simulink model "mcb_microchip_pmsm_autotuner_SAME70"  (R2023a)
settings: Solver=FixedStepDiscrete  StartTime=0.0  StopTime=30  RelTol=1e-3  EnableMultiTasking=on
InitFcn:
  | mcb_microchip_pmsm_autotuner_SAME70_data;
values from neighbouring files (symbols this model uses):
  PU_System = mcb_SetPUSystem(pmsm,inverter)    [mcb_microchip_pmsm_autotuner_SAME70_data.m]
  Ts = T_pwm    (= 5e-05)    [mcb_microchip_pmsm_autotuner_SAME70_data.m]
  Ts_motor = T_pwm/2    (= 2.5e-05)    [mcb_microchip_pmsm_autotuner_SAME70_data.m]
  Ts_simulink = T_pwm/2    (= 2.5e-05)    [mcb_microchip_pmsm_autotuner_SAME70_data.m]
  Ts_speed = 2 * Ts    (= 0.0001)    [mcb_microchip_pmsm_autotuner_SAME70_data.m]
undefined symbols (not defined in the file or in its folder): A24, AD10, AD7, inverter, LQFP144, MaxPer, ms, ns, PA0, PA1, PA10, PA11, PA12, PA13, PA16, PA18, PA9, PB0, PD18, PD19, PD24, PD25, PD26, PI_params, Pin, pmsm, Resol, SAME70Q21B, target, Timer, Unsigned
libraries: simulink x13, MCHP_Blockset x13, mcbcontrolslib x7, slpidlib x3, mcbpositiondecoderlib x3, svdutilitieslib x3, mcbplantlib x1, autolibpmsmexterior x1, focautotunershared x1
(part 3 of 4)

== system mcb_microchip_pmsm_autotuner_SAME70/Microcontroller/Heartbeat LED ==
  Codegen : Subsystem  VariantControl=(codegen)
  Sim : Subsystem  VariantControl=(sim)

== system mcb_microchip_pmsm_autotuner_SAME70/Microcontroller/Input HW Drivers ==
  PhaseCurr_fb : Inport
  Position_fb : Inport  Port=2
  Codegen : Subsystem  VariantControl=(codegen)
  Sim : Subsystem  VariantControl=(sim)
  IabADC : Outport
  VdcADC : Outport  Port=2
  Vabc_ADC : Outport  Port=3
  eQEP : Outport  Port=4

== system mcb_microchip_pmsm_autotuner_SAME70/Microcontroller/Input Scaling ==
  Mode : Inport
  Iab_ADC : Inport  Port=2
  Vdc_ADC : Inport  Port=3
  Vabc_ADC : Inport  Port=4
  Gain : Gain  Gain=inverter.VoltPerCount  OutDataTypeStr=dataType  RndMeth=Simplest
  Gain1 : Gain  Gain=inverter.VoltPerCount  OutDataTypeStr=dataType  RndMeth=Simplest
  Variant Subsystem : Subsystem  Variant=on
  Iab : Outport
  Vdc : Outport  Port=2
  Vabc : Outport  Port=3
  wires:
  Variant Subsystem/1(Iab) -> Iab/1
  Mode/1 -> Variant Subsystem/1(Mode)
  Iab_ADC/1 -> Variant Subsystem/2(Iab_ADC)
  Vdc_ADC/1 -> Gain/1
  Gain/1 -> Vdc/1
  Vabc_ADC/1 -> Gain1/1
  Gain1/1 -> Vabc/1

== system mcb_microchip_pmsm_autotuner_SAME70/Microcontroller/Mode Control ==
  ClosedLoop : Subsystem  VariantControl=inverter.ADCOffsetCalibEnable == 0 && pmsm.QEPIndexPresent == true
  CurrentCalib : Subsystem  VariantControl=inverter.ADCOffsetCalibEnable == 1 && pmsm.QEPIndexPresent == true
  CurrentPosCalib : Subsystem  VariantControl=inverter.ADCOffsetCalibEnable == 1 && pmsm.QEPIndexPresent == false
  PosCalib : Subsystem  VariantControl=inverter.ADCOffsetCalibEnable == 0 && pmsm.QEPIndexPresent == false
  Mode : Outport

== system mcb_microchip_pmsm_autotuner_SAME70/Microcontroller/Output PWM Drivers ==
  PWM_In : Inport
  InvEn : Inport  Port=2
  Codegen : Subsystem  VariantControl=(codegen)
  Sim : Subsystem  VariantControl=(sim)
  PWM : Outport

== system mcb_microchip_pmsm_autotuner_SAME70/Microcontroller/Output Scaling ==
  Mode : Inport
  Vabc_Ref : Inport  Port=2
  InverterEn : Inport  Port=3
  Constant2 : Constant  OutDataTypeStr=dataType
  Current offset measurement : Constant  Value=[0 0 0]  OutDataTypeStr=dataType
  Mode1 : InportShadow
  Mode2 : InportShadow
  Position offset calibration : Constant  Value=[0.2 -0.1 -0.1]  OutDataTypeStr=dataType
  Switch : Switch  Threshold=1  SaturateOnIntegerOverflow=off  InputSameDT=off
  Switch1 : Switch  Threshold=2  SaturateOnIntegerOverflow=off  InputSameDT=off
  Switch2 : Switch  Threshold=2  SaturateOnIntegerOverflow=off  InputSameDT=off
  PWM : Outport
  InvEn : Outport  Port=2
  wires:
  Switch/1 -> PWM/1
  Switch1/1 -> InvEn/1
  Mode/1 -> Switch/2
  Current offset measurement/1 -> Switch/3
  Switch2/1 -> Switch/1
  Mode1/1 -> Switch2/2
  Vabc_Ref/1 -> Switch2/1
  Position offset calibration/1 -> Switch2/3
  InverterEn/1 -> Switch1/1
  Mode2/1 -> Switch1/2
  Constant2/1 -> Switch1/3

== system mcb_microchip_pmsm_autotuner_SAME70/Microcontroller/SCI In Abstraction ==
  SCI_Data : Inport
  Mode : Inport  Port=2
  Variant Subsystem : Subsystem  Variant=on  VariantControlMode=sim codegen switching
  ConfigAndCommand : Outport
  DebugSel : Outport  Port=2
  wires:
  Variant Subsystem/1(ConfigAndCommand) -> ConfigAndCommand/1
  Variant Subsystem/2(DebugSel) -> DebugSel/1
  SCI_Data/1 -> Variant Subsystem/1(SCI_Data)
  Mode/1 -> Variant Subsystem/2(Mode)

== system mcb_microchip_pmsm_autotuner_SAME70/Microcontroller/SCI Out Abstraction ==
  DebugSel : Inport
  DebugData : Inport  Port=2
  Bus Selector : BusSelector  OutputSignals=PI Params.daxis_gains.P,PI Params.daxis_gains.I,PI Params.qaxis_gains.P,PI Params.qaxis_gains.I,PI Params.speed_gains.P,PI Params.speed_gains.I
  Bus Selector1 : BusSelector  OutputSignals=SpeedFb,Iab,Theta
  Byte Pack : svdutilitieslib/Byte Pack  maskPackedDataType=uint8  datatypes={'single'}  byteAlign=1  blockPlatform=tic2000
  Byte Pack1 : svdutilitieslib/Byte Pack  maskPackedDataType=uint8  datatypes={'single'}  byteAlign=1  blockPlatform=tic2000
  Byte Pack2 : svdutilitieslib/Byte Pack  maskPackedDataType=uint8  datatypes={'single'}  byteAlign=1  blockPlatform=tic2000
  Constant : Constant  Value=0  OutDataTypeStr=dataType
  Counter Free-Running : simulink/Sources/Counter Free-Running  NumBits=3  tsamp=0.5
  Data Type Conversion : DataTypeConversion  OutDataTypeStr=single  RndMeth=Simplest  SaturateOnIntegerOverflow=off
  Demux : Demux  Outputs=2
  Multiport Switch : MultiPortSwitch  Inputs=7  DiagnosticForDefault=None  SaturateOnIntegerOverflow=off  InputSameDT=off
  Multiport Switch1 : MultiPortSwitch  Inputs=4  DiagnosticForDefault=None  SaturateOnIntegerOverflow=off  InputSameDT=off
  Mux : Mux  Inputs=3
  Rate Transition2 : RateTransition  Deterministic=off  OutPortSampleTime=Ts
  DebugSignal : Outport
  wires:
  Counter Free-Running/1 -> Data Type Conversion/1
  Data Type Conversion/1 -> Rate Transition2/1
  DebugData/1 -> Bus Selector1/1, Bus Selector/1
  Bus Selector/4 -> Multiport Switch/5  "<I>"
  Bus Selector/5 -> Multiport Switch/6  "<P>"
  Bus Selector/3 -> Multiport Switch/4  "<P>"
  Bus Selector/6 -> Multiport Switch/7  "<I>"
  Bus Selector/2 -> Multiport Switch/3  "<I>"
  Bus Selector/1 -> Multiport Switch/2  "<P>"
  Constant/1 -> Multiport Switch/8
  DebugSel/1 -> Multiport Switch1/1
  Multiport Switch/1 -> Byte Pack/1
  Multiport Switch1/1 -> Byte Pack1/1
  Bus Selector1/1 -> Multiport Switch1/2  "<SpeedFb>"
  Bus Selector1/3 -> Multiport Switch1/5  "<Theta>"
  Bus Selector1/2 -> Demux/1  "<Iab>"
  Demux/1 -> Multiport Switch1/3
  Demux/2 -> Multiport Switch1/4
  Mux/1 -> DebugSignal/1
  Rate Transition2/1 -> Multiport Switch/1, Byte Pack2/1
  Byte Pack/1 -> Mux/2
  Byte Pack1/1 -> Mux/3
  Byte Pack2/1 -> Mux/1

== system mcb_microchip_pmsm_autotuner_SAME70/Microcontroller/SCI_Rx ==
  CodeGen : Subsystem
  Sim : Subsystem
  Variant Source : VariantSource  VariantControlMode=sim codegen switching
  Data : Outport
  wires:
  CodeGen/1(Data) -> Variant Source/1
  Variant Source/1 -> Data/1
  Sim/1(Data) -> Variant Source/2

== system mcb_microchip_pmsm_autotuner_SAME70/Microcontroller/SCI_Tx ==
  SCI_Tx_Data : Inport
  Codegen : Subsystem  SystemSampleTime=0.03  VariantControl=(codegen)
  Sim : Subsystem  VariantControl=(sim)

== system mcb_microchip_pmsm_autotuner_SAME70/Inverter and Motor/Inverter and Motor/Codegen ==
  Duty_Cycles : Inport
  Ground : Ground
  Terminator : Terminator
  PhaseCurr_fb : Outport
  Position_fb : Outport  Port=2
  wires:
  Duty_Cycles/1 -> Terminator/1
  Ground/1 -> PhaseCurr_fb/1, Position_fb/1

== system mcb_microchip_pmsm_autotuner_SAME70/Inverter and Motor/Inverter and Motor/Sim ==
  Duty_Cycles : Inport
  Motor : Subsystem
  RT1 : RateTransition  Deterministic=off  OutPortSampleTime=Ts_simulink
  RT2 : RateTransition  Deterministic=off  OutPortSampleTime=Ts_simulink
  Rate Transition2 : RateTransition  Deterministic=off  OutPortSampleTime=Ts
  Rate Transition3 : RateTransition  Deterministic=off  OutPortSampleTime=Ts_inverter
  Rate Transition4 : RateTransition  Deterministic=off  OutPortSampleTime=Ts
  Sensor Measurements : Subsystem
  PhaseCurr_fb : Outport
  Position_fb : Outport  Port=2
  wires:
  RT1/1 -> Sensor Measurements/2(PhaseCurr)
  Duty_Cycles/1 -> Rate Transition3/1
  Sensor Measurements/2(Position_fb) -> Rate Transition4/1
  Sensor Measurements/1(PhaseCurr_fb) -> Rate Transition2/1
  Rate Transition2/1 -> PhaseCurr_fb/1
  Rate Transition4/1 -> Position_fb/1
  RT2/1 -> Sensor Measurements/1(Info)
  Rate Transition3/1 -> Motor/1(Duty_Cycles)
  Motor/1(ThetaMech) -> RT2/1
  Motor/2(Iabc) -> RT1/1

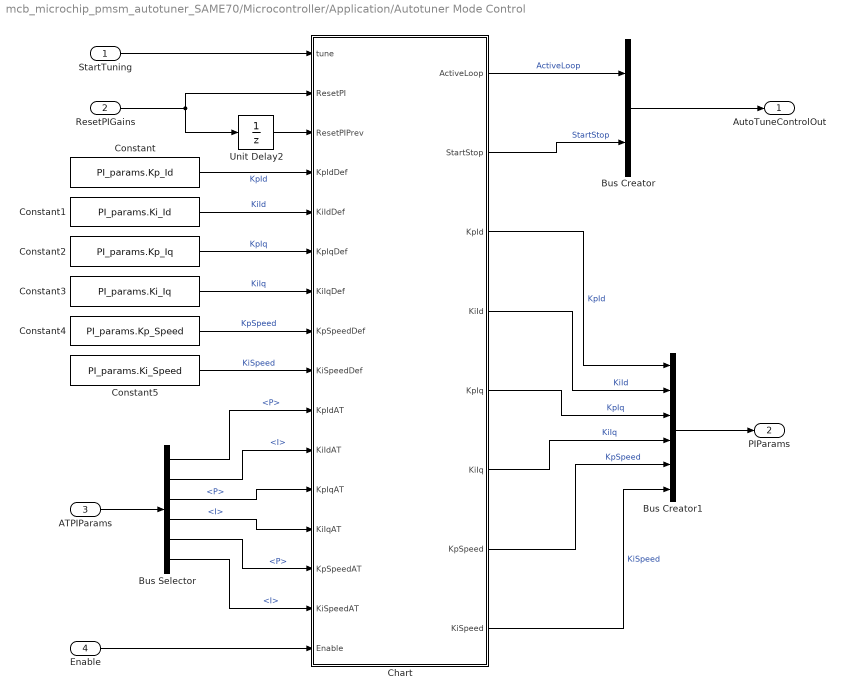
== system mcb_microchip_pmsm_autotuner_SAME70/Microcontroller/Application/Autotuner Mode Control ==
  StartTuning : Inport
  ResetPIGains : Inport  Port=2
  ATPIParams : Inport  Port=3
  Enable : Inport  Port=4
  Bus Creator : BusCreator  Inputs=2
  Bus Creator1 : BusCreator  Inputs=6
  Bus Selector : BusSelector  OutputSignals=daxis_gains.P,daxis_gains.I,qaxis_gains.P,qaxis_gains.I,speed_gains.P,speed_gains.I
  Chart : Stateflow chart  TreatAsAtomicUnit=on
      settings: PortSchema="{\"entries\":[{\"content\":{\"sides\":[{\"content\":{\"connectorIds\":[\"In1\",\"In2\",\"In3\",\"In11\",\"In5\",\"In13\",\"In7\",\"In15\",\"In9\",\"In10\",\"In4\",\"In12\",\"In6\",\"In14\",\"In8\",\"In16\"]},\"type\":\"ConnectorPlacement.EquallySpacedRectSide\",\"uuid\":\"db330f04-e99e-4301-937c-d4ce54467736\"},{\"content\":{\"connectorIds\":[\"Out1\",\"Out2\",\"Out6\",\"Out3\",\"Out7\",\"Out4\",\"Out8\",\"Out5\"],\"side\":\"RIGHT\"},\"type\":\"ConnectorPlacement.EquallySpacedRectSide\",\"uuid\":\"9e1eb776-face-44e3-b5c8-2bc4aae2d103\"},{\"content\":{\"side\":\"TOP\"},\"type\":\"ConnectorPlacement.EquallySpacedRectSide\",\"uuid\":\"fe7f5f84-3794-4c11-8654-00d868fc153d\"}]},\"type\":\"ConnectorPlacement.EquallySpacedConnector\",\"uuid\":\"80e686bd-7f62-451d-a5b9-48803e23a29a\"}],\"packageUris\":[\"http://schema.mathworks.com/mf0/Connector/R2020b\"],\"version\":\"1.0\"}"
  Constant : Constant  Value=PI_params.Kp_Id  OutDataTypeStr=dataType
  Constant1 : Constant  Value=PI_params.Ki_Id  OutDataTypeStr=dataType
  Constant2 : Constant  Value=PI_params.Kp_Iq  OutDataTypeStr=dataType
  Constant3 : Constant  Value=PI_params.Ki_Iq  OutDataTypeStr=dataType
  Constant4 : Constant  Value=PI_params.Kp_Speed  OutDataTypeStr=dataType
  Constant5 : Constant  Value=PI_params.Ki_Speed  OutDataTypeStr=dataType
  Unit Delay2 : UnitDelay  SampleTime=-1  HasFrameUpgradeWarning=on
  AutoTuneControlOut : Outport
  PIParams : Outport  Port=2
  wires:
  Chart/2(StartStop) -> Bus Creator/2  "StartStop"
  Chart/1(ActiveLoop) -> Bus Creator/1  "ActiveLoop"
  StartTuning/1 -> Chart/1(tune)
  Bus Creator/1 -> AutoTuneControlOut/1
  ResetPIGains/1 -> Unit Delay2/1, Chart/2(ResetPI)
  Unit Delay2/1 -> Chart/3(ResetPIPrev)
  Bus Creator1/1 -> PIParams/1
  Constant/1 -> Chart/11(KpIdDef)  "KpId"
  Constant1/1 -> Chart/5(KiIdDef)  "KiId"
  Constant2/1 -> Chart/13(KpIqDef)  "KpIq"
  Constant3/1 -> Chart/7(KiIqDef)  "KiIq"
  Constant4/1 -> Chart/15(KpSpeedDef)  "KpSpeed"
  Constant5/1 -> Chart/9(KiSpeedDef)  "KiSpeed"
  ATPIParams/1 -> Bus Selector/1
  Chart/3(KiId) -> Bus Creator1/2  "KiId"
  Chart/6(KpId) -> Bus Creator1/1  "KpId"
  Chart/4(KiIq) -> Bus Creator1/4  "KiIq"
  Chart/5(KiSpeed) -> Bus Creator1/6  "KiSpeed"
  Chart/8(KpSpeed) -> Bus Creator1/5  "KpSpeed"
  Chart/7(KpIq) -> Bus Creator1/3  "KpIq"
  Bus Selector/1 -> Chart/10(KpIdAT)  "<P>"
  Bus Selector/2 -> Chart/4(KiIdAT)  "<I>"
  Bus Selector/3 -> Chart/12(KpIqAT)  "<P>"
  Bus Selector/4 -> Chart/6(KiIqAT)  "<I>"
  Bus Selector/5 -> Chart/14(KpSpeedAT)  "<P>"
  Bus Selector/6 -> Chart/8(KiSpeedAT)  "<I>"
  Enable/1 -> Chart/16(Enable)

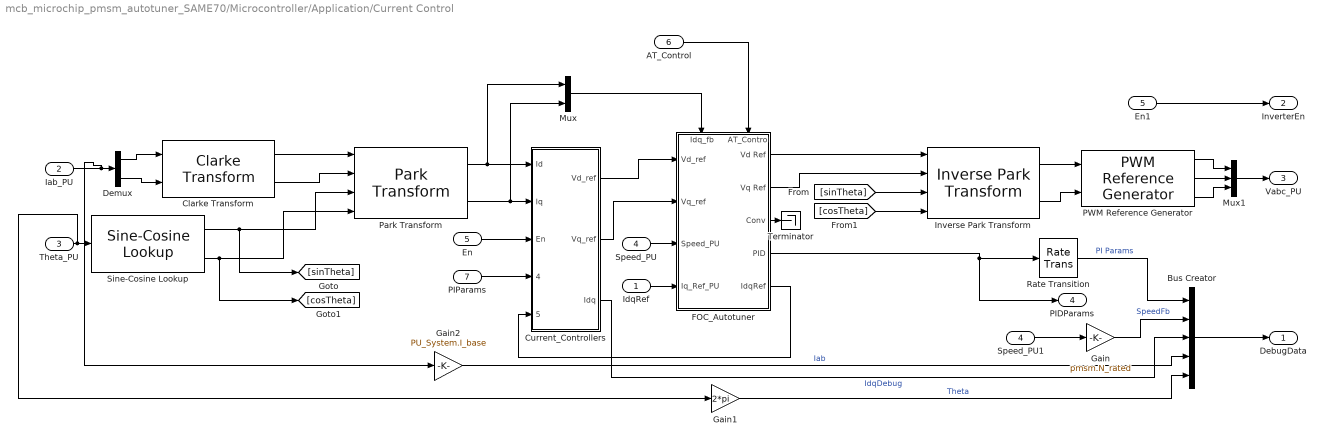
== system mcb_microchip_pmsm_autotuner_SAME70/Microcontroller/Application/Current Control ==
  IdqRef : Inport
  Iab_PU : Inport  Port=2
  Theta_PU : Inport  Port=3
  Speed_PU : Inport  Port=4
  En : Inport  Port=5
  AT_Control : Inport  Port=6
  PIParams : Inport  Port=7
  Bus Creator : BusCreator  Inputs=5
  Clarke Transform : mcbcontrolslib/Clarke Transform  VariantControl=Variant2
      settings: LibrarySourceBlock=mcblib/Controls/Math Transforms/Clarke Transform
  Current_Controllers : Subsystem
  Demux : Demux  Outputs=2
  En1 : InportShadow  Port=5
  FOC_Autotuner : Subsystem
      settings: PortSchema="{\"entries\":[{\"content\":{\"sides\":[{\"content\":{\"connectorIds\":[\"In1\",\"In2\",\"In3\",\"In4\"]},\"type\":\"ConnectorPlacement.EquallySpacedRectSide\",\"uuid\":\"d78fff67-8aa2-4207-86fb-3e88b10df8de\"},{\"content\":{\"connectorIds\":[\"Out1\",\"Out2\",\"Out3\",\"Out4\",\"Out5\"],\"side\":\"RIGHT\"},\"type\":\"ConnectorPlacement.EquallySpacedRectSide\",\"uuid\":\"bf301153-8c5c-4ae3-9b8a-c1a5f30f46e2\"},{\"content\":{\"connectorIds\":[\"In5\",\"In6\"],\"side\":\"TOP\"},\"type\":\"ConnectorPlacement.EquallySpacedRectSide\",\"uuid\":\"3bbd5c92-46d9-4f27-a433-e7f98646a58a\"},{\"content\":{\"side\":\"BOTTOM\"},\"type\":\"ConnectorPlacement.EquallySpacedRectSide\",\"uuid\":\"b65b8459-786f-43ba-a835-654a4f56e2f9\"}]},\"type\":\"ConnectorPlacement.EquallySpacedConnector\",\"uuid\":\"e56590db-8f28-412e-a603-6147134707c4\"}],\"packageUris\":[\"http://schema.mathworks.com/mf0/Connector/R2020b\"],\"version\":\"1.0\"}"
  Gain : Gain  Gain=pmsm.N_rated  RndMeth=Simplest  OutDataTypeStr=Inherit: Same as input
  Gain1 : Gain  Gain=2*pi  RndMeth=Simplest  OutDataTypeStr=Inherit: Same as input
  Gain2 : Gain  Gain=PU_System.I_base  RndMeth=Simplest  OutDataTypeStr=Inherit: Same as input
  Inverse Park Transform : mcbcontrolslib/Inverse Park Transform  AxisAlignment=D-axis
      settings: LibrarySourceBlock=mcblib/Controls/Math Transforms/Inverse Park Transform
  Mux : Mux  Inputs=2
  Mux1 : Mux  Inputs=3
  PWM Reference Generator : mcbcontrolslib/PWM Reference Generator  inSignal=Valphabeta  modType=SVM: space vector modulation
      settings: LibrarySourceBlock=mcblib/Controls/Math Transforms/PWM Reference Generator
  Park Transform : mcbcontrolslib/Park Transform  AxisAlignment=D-axis
      settings: LibrarySourceBlock=mcblib/Controls/Math Transforms/Park Transform
  Rate Transition : RateTransition  Deterministic=off  OutPortSampleTime=Ts
  Sine-Cosine Lookup : mcbcontrolslib/Sine-Cosine Lookup  AngleInput=Per-unit  N_points=1024
      settings: LibrarySourceBlock=mcblib/Controls/Math Transforms/Sine-Cosine Lookup
  Speed_PU1 : InportShadow  Port=4
  Terminator : Terminator
  DebugData : Outport
  InverterEn : Outport  Port=2
  Vabc_PU : Outport  Port=3
  PIDParams : Outport  Port=4
  wires:
  Demux/1 -> Clarke Transform/1
  Demux/2 -> Clarke Transform/2
  Clarke Transform/1 -> Park Transform/1
  Clarke Transform/2 -> Park Transform/2
  Theta_PU/1 -> Gain1/1, Sine-Cosine Lookup/1
  Sine-Cosine Lookup/1 -> Park Transform/3, [sinTheta]
  Sine-Cosine Lookup/2 -> Park Transform/4, [cosTheta]
  Park Transform/1 -> Mux/1, Current_Controllers/1(Id)
  Park Transform/2 -> Mux/2, Current_Controllers/2(Iq)
  En/1 -> Current_Controllers/3(En)
  Current_Controllers/1(Vd_ref) -> FOC_Autotuner/1(Vd_ref)
  Current_Controllers/2(Vq_ref) -> FOC_Autotuner/2(Vq_ref)
  Speed_PU/1 -> FOC_Autotuner/3(Speed_PU)
  Mux/1 -> FOC_Autotuner/5(Idq_fb)
  IdqRef/1 -> FOC_Autotuner/4(Iq_Ref_PU)
  FOC_Autotuner/5(IdqRef) -> Current_Controllers/5(Idq_Ref)
  AT_Control/1 -> FOC_Autotuner/6(AT_Control)
  FOC_Autotuner/1(Vd Ref) -> Inverse Park Transform/1
  FOC_Autotuner/2(Vq Ref) -> Inverse Park Transform/2
  [sinTheta] -> Inverse Park Transform/3
  [cosTheta] -> Inverse Park Transform/4
  Inverse Park Transform/1 -> PWM Reference Generator/1
  Inverse Park Transform/2 -> PWM Reference Generator/2
  PWM Reference Generator/1 -> Mux1/1
  PWM Reference Generator/2 -> Mux1/2
  PWM Reference Generator/3 -> Mux1/3
  Mux1/1 -> Vabc_PU/1
  En1/1 -> InverterEn/1
  PIParams/1 -> Current_Controllers/4(PIParams)
  FOC_Autotuner/3(Conv) -> Terminator/1
  FOC_Autotuner/4(PID) -> PIDParams/1, Rate Transition/1
  Bus Creator/1 -> DebugData/1
  Rate Transition/1 -> Bus Creator/1  "PI Params"
  Speed_PU1/1 -> Gain/1
  Gain/1 -> Bus Creator/2  "SpeedFb"
  Current_Controllers/3(Idq) -> Bus Creator/3  "IdqDebug"
  Iab_PU/1 -> Gain2/1, Demux/1
  Gain1/1 -> Bus Creator/5  "Theta"
  Gain2/1 -> Bus Creator/4  "Iab"

== system mcb_microchip_pmsm_autotuner_SAME70/Microcontroller/Application/Speed Control ==
  SpeedRef : Inport
  Enable : Inport  Port=2
  Speed_Meas_PU : Inport  Port=3
  EnClosedLoop : Inport  Port=4
  PIParams : Inport  Port=5
  EnClosedLoop1 : InportShadow  Port=4
  Gain : Gain  Gain=1/pmsm.N_rated  RndMeth=Simplest  OutDataTypeStr=Inherit: Same as input
  PI_Controller_Speed : Subsystem
  Rate Limiter : RateLimiter  RisingSlewLimit=10  FallingSlewLimit=-10  SampleTimeMode=inherited
  Switch : Switch  Criteria=u2 > Threshold  SaturateOnIntegerOverflow=off  InputSameDT=off
  IdqRef_PU : Outport  VectorParamsAs1DForOutWhenUnconnected=off
  wires:
  PI_Controller_Speed/1(Iq_ref) -> IdqRef_PU/1
  SpeedRef/1 -> Gain/1
  Speed_Meas_PU/1 -> Switch/3, PI_Controller_Speed/2(N_fb)  "Speed_fb"
  Enable/1 -> PI_Controller_Speed/3(Enable)
  EnClosedLoop/1 -> PI_Controller_Speed/4(EnClosedLoop)
  Gain/1 -> Switch/1
  Switch/1 -> Rate Limiter/1
  Rate Limiter/1 -> PI_Controller_Speed/1(N_ref)  "Speed_Ref"
  EnClosedLoop1/1 -> Switch/2
  PIParams/1 -> PI_Controller_Speed/5(PIParams)

== system mcb_microchip_pmsm_autotuner_SAME70/Microcontroller/Application Abstraction/Variant Subsystem ==
  eQEPCnt : Inport
  eQEPIndex : Inport  Port=2
  Mode : Inport  Port=3
  Index Absent : Subsystem  VariantControl=pmsm.QEPIndexPresent == false
  Index Present : Subsystem  VariantControl=pmsm.QEPIndexPresent == true
  Theta : Outport
  Speed : Outport  Port=2
  EnClosedLoop : Outport  Port=3

== system mcb_microchip_pmsm_autotuner_SAME70/Microcontroller/Heartbeat LED/Codegen ==
  DBG LED 1 : MCHP_Blockset/Digital IO/Digital Output Write  PORT=Dynamic Options  PORT_TXT="C   [ 0 : 31 ]"  PIN=23  PACK=off  SIMULTANEOUS=off  ORDERING=None  SampleTime=-1  MCHP_PORT={Digital Out}{DOU}1:1:C23;  MCHP_MASTERLINK=mcb_microchip_pmsm_autotuner_SAME70/Microcontroller/Configurations/Microchip Master
      settings: SourceProductName=MPLAB Device Blocks for Simulink
  Delay 10Hz : Delay  DelayLength=1  InitialCondition=0  SampleTime=0.25
  Logical Operator : Logic  Operator=NOT  AllPortsSameDT=off  OutDataTypeStr=boolean
  wires:
  Delay 10Hz/1 -> Logical Operator/1
  Logical Operator/1 -> DBG LED 1/1, Delay 10Hz/1

== system mcb_microchip_pmsm_autotuner_SAME70/Microcontroller/Heartbeat LED/Sim ==

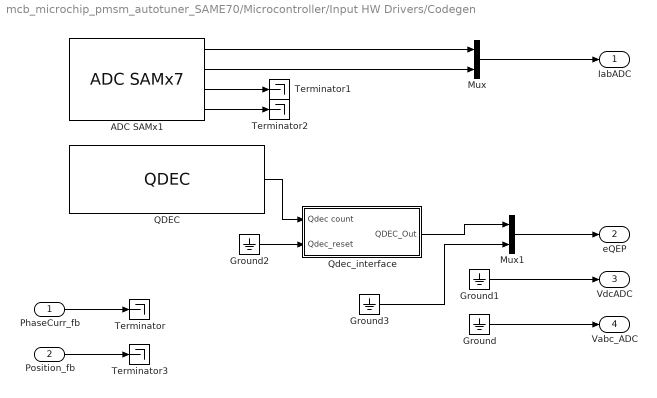
== system mcb_microchip_pmsm_autotuner_SAME70/Microcontroller/Input HW Drivers/Codegen ==
  PhaseCurr_fb : Inport
  Position_fb : Inport  Port=2
  ADC SAMx1 : MCHP_Blockset/Analog IO/ADC SAMx7  Priority=-2000  AFECx=AFE Controller 0  SIGNMODE_SingleEnded=Unsigned (uint16)  SIGNMODE_Differential=Unsigned (uint16)  AFEC0_seq0=Dynamic Options  AFEC0_seq0_TXT="AD0 / PD30   &   AD6 / PA17"  AFEC1_seq0=Dynamic Options  AFEC1_seq0_TXT=Not used  AFEC0_seq1=Dynamic Options  AFEC0_seq1_TXT=AD7 / PA18  AFEC1_seq1=Dynamic Options  AFEC1_seq1_TXT=Not used  AFEC0_seq2=Dynamic Options  AFEC0_seq2_TXT=AD10 / PB0  AFEC1_seq2=Dynamic Options  AFEC1_seq2_TXT=Not used  AFEC0_seq3=Dynamic Options  AFEC0_seq3_TXT=Not used  AFEC1_seq3=Dynamic Options  AFEC1_seq3_TXT=Not used  AFEC0_seq4=Dynamic Options  AFEC0_seq4_TXT=Not used  AFEC1_seq4=Dynamic Options  AFEC1_seq4_TXT=Not used  AFEC0_seq5=Dynamic Options  AFEC0_seq5_TXT=Not used  AFEC1_seq5=Dynamic Options  AFEC1_seq5_TXT=Not used  AFEC0_seq6=Dynamic Options  AFEC0_seq6_TXT=Not used  AFEC1_seq6=Dynamic Options  AFEC1_seq6_TXT=Not used  AFEC0_seq7=Dynamic Options  AFEC0_seq7_TXT=Not used  AFEC1_seq7=Dynamic Options  AFEC1_seq7_TXT=Not used  AFEC0_seq8=Dynamic Options  AFEC0_seq8_TXT=Not used  AFEC1_seq8=Dynamic Options  AFEC1_seq8_TXT=Not used  AFEC0_seq9=Dynamic Options  AFEC0_seq9_TXT=Not used  AFEC1_seq9=Dynamic Options  AFEC1_seq9_TXT=Not used  AFEC0_seq10=Dynamic Options  AFEC0_seq10_TXT=Not used  AFEC1_seq10=Dynamic Options  AFEC1_seq10_TXT=Not used  AFEC0_seq11=Dynamic Options  AFEC0_seq11_TXT=Not used  AFEC1_seq11=Dynamic Options  AFEC1_seq11_TXT=Not used  SampleTime=Ts  S_INPUT=[-1]  S_INPUT_Size=[3]  S_OUTPUT=[]  S_OUTPUT_Size=[]  S_ListCustomDatatype=S.S_ListCustomDatatype={};  MCHP_AFECC_CLOCK_REQUEST=''  MCHP_AFECC_CLOCK_RESULT=''  MCHP_USER_INTERRUPTS=0  MCHP_PORT={AD0 AFEC0}{AD0}15:2:P126;{AD6 AFEC0}{AD6}15:2:P17;{AD7 AFEC0}{AD7}15:2:P18;{AD10 AFEC0}{AD10}15:2:P32;  MCHP_MASTERLINK=mcb_microchip_pmsm_autotuner_SAME70/Microcontroller/Configurations/Microchip Master  Rin=< 200 Ohm  RES=12-bit Standard  AFEC0_Synchronisation=Triggered by user defined source  AFEC0_Trig=PWM0 event line 0  AFEC0_TrigTimeStep=on  AFEC1_Synchronisation=Triggered by user defined source  AFEC1_Trig=PWM1 event line 0  AFEC1_TrigTimeStep=off  ADC_TrigInfo=0  AFEC0_seq0_GAIN=1  AFEC1_seq0_GAIN=1  AFEC0_seq1_GAIN=1  AFEC1_seq1_GAIN=1  AFEC0_seq2_GAIN=1  AFEC1_seq2_GAIN=1  AFEC0_seq3_GAIN=1  AFEC1_seq3_GAIN=1  AFEC0_seq4_GAIN=1  AFEC1_seq4_GAIN=1  AFEC0_seq5_GAIN=1  AFEC1_seq5_GAIN=1  AFEC0_seq6_GAIN=1  AFEC1_seq6_GAIN=1  AFEC0_seq7_GAIN=1  AFEC1_seq7_GAIN=1  AFEC0_seq8_GAIN=1  AFEC1_seq8_GAIN=1  AFEC0_seq9_GAIN=1  AFEC1_seq9_GAIN=1  AFEC0_seq10_GAIN=1  AFEC1_seq10_GAIN=1  AFEC0_seq11_GAIN=1  AFEC1_seq11_GAIN=1  AFEC0_seq0_OFFSET=0  AFEC1_seq0_OFFSET=0  AFEC0_seq1_OFFSET=0  AFEC1_seq1_OFFSET=0  AFEC0_seq2_OFFSET=0  AFEC1_seq2_OFFSET=0  AFEC0_seq3_OFFSET=0  AFEC1_seq3_OFFSET=0  AFEC0_seq4_OFFSET=0  AFEC1_seq4_OFFSET=0  AFEC0_seq5_OFFSET=0  AFEC1_seq5_OFFSET=0  AFEC0_seq6_OFFSET=0  AFEC1_seq6_OFFSET=0  AFEC0_seq7_OFFSET=0  AFEC1_seq7_OFFSET=0  AFEC0_seq8_OFFSET=0  AFEC1_seq8_OFFSET=0  AFEC0_seq9_OFFSET=0  AFEC1_seq9_OFFSET=0  AFEC0_seq10_OFFSET=0  AFEC1_seq10_OFFSET=0  AFEC0_seq11_OFFSET=0  AFEC1_seq11_OFFSET=0
      settings: SourceProductName=MPLAB Device Blocks for Simulink
  Ground{,1..3} (4 alike) : Ground
  Mux : Mux  Inputs=2
  Mux1 : Mux  Inputs=2
  QDEC : MCHP_Blockset/QEI/QDEC  QDEC_REF=Dynamic Options  QDEC_REF_TXT=TC0  PHA_PIN=Dynamic Options  PHA_PIN_TXT=PA0 / Pin[102]  PHB_PIN=Dynamic Options  PHB_PIN_TXT=PA1 / Pin[99]  IDX_PIN=Dynamic Options  IDX_PIN_TXT=PA16 / Pin[45]  INVERT_PHA=off  INVERT_PHB=off  INVERT_IDX=off  SWAP_PHA_PHB=off  SampleTime=Ts  MCHP_PORT={TC0}{TIOA0}3:0:P0;{TC0}{TIOB0}3:0:P1;{TC0}{TIOB1}3:0:P16;  MCHP_MASTERLINK=mcb_microchip_pmsm_autotuner_SAME70/Microcontroller/Configurations/Microchip Master  MCHP_TIMER_REQUEST={Quadrature Decoder (Phase Counter)}{QDEC0}20:4:4:0:[1]:65535;{Quadrature Decoder (IDX Counter)}{QDEC0}20:4:4:0:[2]:65535;{Quadrature Decoder (Speed Measurement Time Base)}{QDEC0}20:4:4:0:[3]:65535;  MCHP_TIMER_RESULT=[1 65535]  QDEC_MODE=Position  POSITION_OUTPUT=is a 16 bits unsigned block output  INDEX_OUTPUT=is not a block output  RESET_INPUT=off  POSITION_RESET_MODE=never reset position  RESET_EDGE=rising edge  POSITION_RESET_VALUE=65535  SPEED_TIME_BASE=Dynamic Options  SPEED_TIME_BASE_TXT=Resol: 53.33(ns) - MaxPer: 3.5(ms)  SPEED_OUTPUT=is a 16 bits unsigned block output  DIR_OUTPUT=is not a block output  DIRCHG_OUTPUT=is not a block output  AUTO_CORRECTION=off  MAX_PERIOD_FILTER=Dynamic Options  MAX_PERIOD_FILTER_TXT=420(ns)  MAXCMP=disabled  MPE_OUTPUT=is not a block output  QERR_OUTPUT=is not a block output
      settings: SourceProductName=MPLAB Device Blocks for Simulink
  Qdec_interface : Subsystem  mask{EnCountPerRev=pmsm.QEPSlits*4}
      mask prompts: EnCountPerRev "Encoder counts per rev"
  Terminator{,1..3} (4 alike) : Terminator
  IabADC : Outport
  eQEP : Outport  Port=2
  VdcADC : Outport  Port=3
  Vabc_ADC : Outport  Port=4
  wires:
  ADC SAMx1/4 -> Terminator2/1
  ADC SAMx1/3 -> Terminator1/1
  Ground2/1 -> Qdec_interface/2(Qdec_reset)
  QDEC/1 -> Qdec_interface/1(Qdec count)
  PhaseCurr_fb/1 -> Terminator/1
  Position_fb/1 -> Terminator3/1
  Ground/1 -> Vabc_ADC/1
  Ground1/1 -> VdcADC/1
  ADC SAMx1/1 -> Mux/1
  ADC SAMx1/2 -> Mux/2
  Mux/1 -> IabADC/1
  Qdec_interface/1(QDEC_Out) -> Mux1/1
  Mux1/1 -> eQEP/1
  Ground3/1 -> Mux1/2

== system mcb_microchip_pmsm_autotuner_SAME70/Microcontroller/Input HW Drivers/Sim ==
  PhaseCurr_fb : Inport
  Position_fb : Inport  Port=2
  Ground : Ground
  Ground1 : Ground
  IabADC : Outport
  eQEP : Outport  Port=2
  VdcADC : Outport  Port=3
  Vabc_ADC : Outport  Port=4
  wires:
  PhaseCurr_fb/1 -> IabADC/1
  Position_fb/1 -> eQEP/1
  Ground/1 -> Vabc_ADC/1
  Ground1/1 -> VdcADC/1

== system mcb_microchip_pmsm_autotuner_SAME70/Microcontroller/Input Scaling/Variant Subsystem ==
  Mode : Inport
  Iab_ADC : Inport  Port=2
  Automatic offset calibration : Subsystem  VariantControl=inverter.ADCOffsetCalibEnable == 1
  Offser via parameter : Subsystem  VariantControl=inverter.ADCOffsetCalibEnable == 0
  Iab : Outport

== system mcb_microchip_pmsm_autotuner_SAME70/Microcontroller/Mode Control/ClosedLoop ==
  Constant : Constant  Value=2  OutDataTypeStr=single  SampleTime=0.1
  Mode : Outport
  wires:
  Constant/1 -> Mode/1

== system mcb_microchip_pmsm_autotuner_SAME70/Microcontroller/Mode Control/CurrentCalib ==
  Step : Step  After=2  OutDataTypeStr=single  SampleTime=0.1
  Mode : Outport
  wires:
  Step/1 -> Mode/1

== system mcb_microchip_pmsm_autotuner_SAME70/Microcontroller/Mode Control/CurrentPosCalib ==
  Add : Sum
  Step : Step  OutDataTypeStr=single  SampleTime=0.1
  Step1 : Step  Time=2  OutDataTypeStr=single  SampleTime=0.1
  Mode : Outport
  wires:
  Step/1 -> Add/1
  Step1/1 -> Add/2
  Add/1 -> Mode/1

== system mcb_microchip_pmsm_autotuner_SAME70/Microcontroller/Mode Control/PosCalib ==
  Step : Step  Before=1  After=2  OutDataTypeStr=single  SampleTime=0.1
  Mode : Outport
  wires:
  Step/1 -> Mode/1

== system mcb_microchip_pmsm_autotuner_SAME70/Microcontroller/Output PWM Drivers/Codegen ==
  PWM_In : Inport
  InvEn : Inport  Port=2
  Constant : Constant  Value=0xF000F  OutDataTypeStr=uint32  SampleTime=-1
  Constant1 : Constant  Value=0  OutDataTypeStr=uint32  SampleTime=-1
  Constant2 : Constant  Value=0  OutDataTypeStr=uint32  SampleTime=-1
  Data Type Conversion : DataTypeConversion  OutDataTypeStr=single  SaturateOnIntegerOverflow=off  RndMeth=Floor
  Ground : Ground
  InvEn1 : InportShadow  Port=2
  Mux3 : Mux  Inputs=3
  PWM SAM7x : MCHP_Blockset/PWM IO/PWM SAM7x  Priority=-2000  PWMx=PWM Controller 0  MaxPeriod_s=Ts  PWM0_pinH0=Dynamic Options  PWM0_pinH0_TXT=PA11 / Pin[64]  PWM0_pinL0=Dynamic Options  PWM0_pinL0_TXT=PD24 / Pin[55]  PWM0_pinH1=Dynamic Options  PWM0_pinH1_TXT=PA12 / Pin[68]  PWM0_pinL1=Dynamic Options  PWM0_pinL1_TXT=PD25 / Pin[52]  PWM0_pinH2=Dynamic Options  PWM0_pinH2_TXT=PA13 / Pin[42]  PWM0_pinL2=Dynamic Options  PWM0_pinL2_TXT=PD26 / Pin[53]  PWM0_pinH3=Dynamic Options  PWM0_pinH3_TXT=Not Used  PWM0_pinL3=Dynamic Options  PWM0_pinL3_TXT=Not Used  PWM1_pinH0=Dynamic Options  PWM1_pinH0_TXT=Not Used  PWM1_pinL0=Dynamic Options  PWM1_pinL0_TXT=Not Used  PWM1_pinH1=Dynamic Options  PWM1_pinH1_TXT=Not Used  PWM1_pinL1=Dynamic Options  PWM1_pinL1_TXT=Not Used  PWM1_pinH2=Dynamic Options  PWM1_pinH2_TXT=Not Used  PWM1_pinL2=Dynamic Options  PWM1_pinL2_TXT=Not Used  PWM1_pinH3=Dynamic Options  PWM1_pinH3_TXT=Not Used  PWM1_pinL3=Dynamic Options  PWM1_pinL3_TXT=Not Used  PWM_Centered=on  PWM_SyncWithPWM0=on  PushPull_Mode=off  SampleTime=Ts  S_INPUT=[-1]  S_INPUT_Size=[3]  S_OUTPUT=[]  S_OUTPUT_Size=[]  S_ListCustomDatatype=S.S_ListCustomDatatype={};  evalin_ws=PWM0max0=MCHP_Fun.Hex2num('40AD4C0000000000');PWM1max0=MCHP_Fun.Hex2num('40AD4C0000000000');PWM2max0=MCHP_Fun.Hex2num('40AD4C0000000000');  MCHP_PWMC_CLOCK_REQUEST=''  MCHP_PWMC_CLOCK_RESULT=''  MCHP_USER_INTERRUPTS=0  MCHP_PORT={PWM0H0 }{PWMH0}4:1:P11;{PWM0L0 }{PWML0}4:1:P120;{PWM0H1 }{PWMH1}4:1:P12;{PWM0L1 }{PWML1}4:1:P121;{PWM0H2 }{PWMH2}4:1:P13;{PWM0L2 }{PWML2}4:1:P122;  MCHP_MASTERLINK=mcb_microchip_pmsm_autotuner_SAME70/Microcontroller/Configurations/Microchip Master  invert_PWMH0=off  invert_PWML0=off  invert_PWMH1=off  invert_PWML1=off  invert_PWMH2=off  invert_PWML2=off  invert_PWMH3=off  invert_PWML3=off  InitPeriod_s=Ts  InitDutyCycle_s=0  InitDeadTimeH_s=1e-6  InitDeadTimeL_s=1e-6  InitEventLine0_ComparatorValue_s=1e-7  InitEventLine1_ComparatorValue_s=[]  BlockInput_VectorScalar=Vectors (grouped by function)  BlockInput_Period=Not a block input  BlockInput_DutyCycle=a Floating Point input within range [-1 1]  BlockInput_DeadTime=Not a block input  BlockInput_OutputOverride=Not a block input  Fault_FPV0=Not forced  Fault_FPV1=Not forced  Fault_FPV2=Not forced  Fault_FPV3=Not forced  Fault_Input0=does nothing  Fault_Input0_FFIL=off  Fault_Input1=does nothing  Fault_Input1_FFIL=off  Fault_Input2=does nothing  Fault_Input2_FFIL=on  Fault_Input3=does nothing  Fault_Input3_FFIL=off  Fault_Input4=does nothing  Fault_Input4_FFIL=on  Fault_Input5=does nothing  Fault_Input5_FFIL=on  Fault_Input6=does nothing  Fault_Input6_FFIL=on  Fault_Input7=does nothing  Fault_Input7_FFIL=on
      settings: SourceProductName=MPLAB Device Blocks for Simulink
  PWM SAM7x Output Override : MCHP_Blockset/PWM IO/PWM SAM7x  Output Override  Priority=-2000  PWMx=PWM Controller 0  SampleTime=Ts  S_INPUT=[-1]  S_INPUT_Size=[3]  S_OUTPUT=[]  S_OUTPUT_Size=[]  S_ListCustomDatatype=S.S_ListCustomDatatype={};  MCHP_MASTERLINK=mcb_microchip_pmsm_autotuner_SAME70/Microcontroller/Configurations/Microchip Master  Init_PWM_OS=0x0000  Init_PWM_OOV=0x0000  Input_PWM_OS=on  Input_PWM_OS_off=off  Input_PWM_OSS=off  Input_PWM_OSS_off=off  Input_PWM_OSSUPD=off  Input_PWM_OSSUPD_off=off  Input_PWM_OSC=off  Input_PWM_OSC_off=off  Input_PWM_OSCUPD=off  Input_PWM_OSCUPD_off=off  Input_PWM_OOV=on
      settings: SourceProductName=MPLAB Device Blocks for Simulink
  Switch1 : Switch  Threshold=0.5  RndMeth=Simplest  SaturateOnIntegerOverflow=off  InputSameDT=off
  Switch4 : Switch  Threshold=0.5  RndMeth=Simplest  SaturateOnIntegerOverflow=off  InputSameDT=off
  stop : Constant  Value=0  OutDataTypeStr=dataType
  PWM : Outport
  wires:
  Mux3/1 -> Switch4/3
  Switch4/1 -> Data Type Conversion/1
  Data Type Conversion/1 -> PWM SAM7x/1
  stop/1 -> Mux3/3, Mux3/2, Mux3/1
  Ground/1 -> PWM/1
  InvEn/1 -> Switch4/2
  PWM_In/1 -> Switch4/1
  Constant1/1 -> Switch1/1
  Switch1/1 -> PWM SAM7x Output Override/1
  Constant2/1 -> PWM SAM7x Output Override/2
  Constant/1 -> Switch1/3
  InvEn1/1 -> Switch1/2

== system mcb_microchip_pmsm_autotuner_SAME70/Microcontroller/Output PWM Drivers/Sim ==
  PWM_In : Inport
  InvEn : Inport  Port=2
  Mux2 : Mux  Inputs=3
  Subsystem : Subsystem
  Switch1 : Switch  Threshold=0.5  RndMeth=Simplest  SaturateOnIntegerOverflow=off  InputSameDT=off
  stop : Constant  Value=0  OutDataTypeStr=Inherit: Inherit via back propagation
  PWM : Outport
  wires:
  Mux2/1 -> Switch1/3
  stop/1 -> Mux2/1, Mux2/3, Mux2/2
  Subsystem/1(PWM_Duty_Cycles) -> Switch1/1
  Switch1/1 -> PWM/1
  InvEn/1 -> Switch1/2
  PWM_In/1 -> Subsystem/1(PWM_In)

== system mcb_microchip_pmsm_autotuner_SAME70/Microcontroller/SCI In Abstraction/Variant Subsystem ==
  SCI_Data : Inport
  Mode : Inport  Port=2
  Codegen : Subsystem  VariantControl=(codegen)
  Sim : Subsystem  VariantControl=(sim)
  ConfigAndCommand : Outport
  DebugSel : Outport  Port=2

== system mcb_microchip_pmsm_autotuner_SAME70/Microcontroller/SCI_Rx/CodeGen ==
  Data Type Conversion : DataTypeConversion  OutDataTypeStr=uint16  SaturateOnIntegerOverflow=off  RndMeth=Floor
  Subsystem : Subsystem
  Subsystem1 : Subsystem
  UART Rx : MCHP_Blockset/BUS UART/UART Rx  UART_REF=UART 0  Flag_Out=on  Rx_Size_popup=User defined  Rx_Size=1  S_Rx_Size=1  Split=Read all received char  SplitChar=10  OutputDefault_popup=do nothing (end of output vector will be undefined)  OutputDefault=-2  ORDERING=None  SampleTime=0.001  MCHP_MASTERLINK=mcb_microchip_pmsm_autotuner_SAME70/Microcontroller/Configurations/Microchip Master  MCHP_COMPILED_INFO="CompiledSampleTime= [0.0010000000000000000208   0 ];CompiledInportDataTypes=[    ];CompiledInportDataWidth=[];"
      settings: SourceProductName=MPLAB Device Blocks for Simulink
  Data : Outport
  wires:
  UART Rx/1 -> Data Type Conversion/1
  UART Rx/2 -> Subsystem1/1(In1)
  Subsystem1/2(Data out) -> Subsystem/1(In1)
  Subsystem1/1(NewData) -> Subsystem/Enable
  Data Type Conversion/1 -> Subsystem1/Enable
  Subsystem/1(Data) -> Data/1

== system mcb_microchip_pmsm_autotuner_SAME70/Microcontroller/SCI_Rx/Sim ==
  Constant : Constant  OutDataTypeStr=single
  Data : Outport
  wires:
  Constant/1 -> Data/1

== system mcb_microchip_pmsm_autotuner_SAME70/Microcontroller/SCI_Tx/Codegen ==
  SCI_Tx_Data : Inport
  Counter Limited : simulink/Sources/Counter Limited  uplimit=target.SerialFrameSize-1  tsamp=-1
  Data : Subsystem  TreatAsAtomicUnit=on
  End : Subsystem  TreatAsAtomicUnit=on
  If : If  IfExpression=u1 == 0  ElseIfExpressions=u1 == single(target.SerialFrameSize-1)
  Start : Subsystem  TreatAsAtomicUnit=on
  wires:
  If/3 -> Data/Action
  If/2 -> End/Action
  If/1 -> Start/Action
  SCI_Tx_Data/1 -> End/1(Data), Data/1(Data), Start/1(Data)
  Counter Limited/1 -> If/1

== system mcb_microchip_pmsm_autotuner_SAME70/Microcontroller/SCI_Tx/Sim ==
  SCI_Tx_Data : Inport
  Terminator : Terminator
  wires:
  SCI_Tx_Data/1 -> Terminator/1

== system mcb_microchip_pmsm_autotuner_SAME70/Inverter and Motor/Inverter and Motor/Sim/Motor ==
  Duty_Cycles : Inport
  Bus Selector : BusSelector  OutputSignals=MtrPos
  Inverter : Subsystem
  Load_Profile (Torque) : Subsystem
  Rate Transition1 : RateTransition  Deterministic=off  OutPortSampleTime=Ts_motor
  Surface Mount PMSM : autolibpmsmexterior/Surface Mount PMSM  port_config=Torque  sim_type=Discrete  Ts=Ts_motor  FilePath=surfacepmsm_motordata.m  P=pmsm.p  Rs=pmsm.Rs + inverter.R_board  Ldq_=pmsm.Ld  KConstText=Permanent flux linkage constant (lambda_pm):  lambda_pm=pmsm.FluxPM  Ke=159.9771  Kt=1.323  mechanical=[pmsm.J, pmsm.B, 0]  idq0=[0 0]  theta_init=0  omega_init=0  KConst=pmsm.FluxPM  lambda_pm_calc=pmsm.FluxPM  RefBlkName='autolibpmsmexterior/Surface Mount PMSM'  aMode=5  Ldq="[0.00078136  0.00078136]"
  Terminator : Terminator
  ThetaMech : Outport
  Iabc : Outport  Port=2
  wires:
  Bus Selector/1 -> ThetaMech/1  "<MtrPos>"
  Surface Mount PMSM/2 -> Iabc/1  "Iabc"
  Load_Profile (Torque)/1(Load_Trq) -> Rate Transition1/1
  Duty_Cycles/1 -> Inverter/1(Duty_abc)
  Surface Mount PMSM/3 -> Terminator/1
  Surface Mount PMSM/1 -> Bus Selector/1
  Rate Transition1/1 -> Surface Mount PMSM/1
  Inverter/1(Vabc) -> Surface Mount PMSM/2

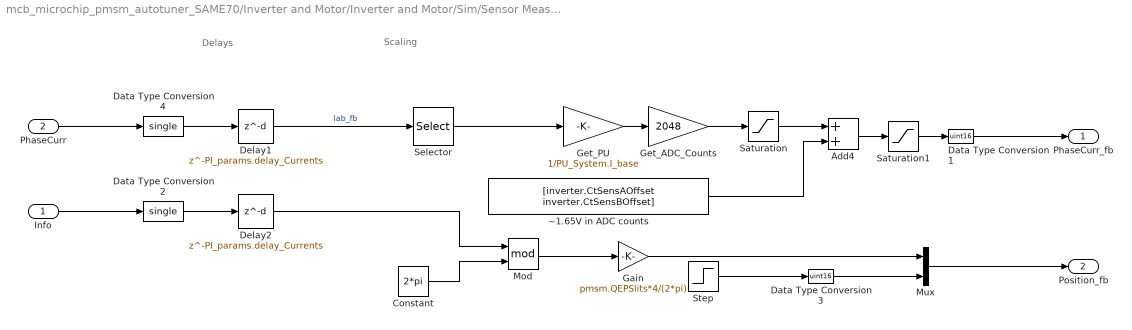
== system mcb_microchip_pmsm_autotuner_SAME70/Inverter and Motor/Inverter and Motor/Sim/Sensor Measurements ==
  note: Scaling
  note: Delays
  Info : Inport
  PhaseCurr : Inport  Port=2
  Add4 : Sum  OutDataTypeStr=uint16
  Constant : Constant  Value=2*pi  OutDataTypeStr=Inherit: Inherit via back propagation  SampleTime=-1
  Data Type Conversion1 : DataTypeConversion  OutDataTypeStr=uint16  SaturateOnIntegerOverflow=off  RndMeth=Floor
  Data Type Conversion2 : DataTypeConversion  OutDataTypeStr=single  RndMeth=Simplest  SaturateOnIntegerOverflow=off
  Data Type Conversion3 : DataTypeConversion  OutDataTypeStr=uint16  SaturateOnIntegerOverflow=off  RndMeth=Floor
  Data Type Conversion4 : DataTypeConversion  OutDataTypeStr=single  RndMeth=Simplest  SaturateOnIntegerOverflow=off
  Delay1 : Delay  DelayLength=PI_params.delay_Currents
  Delay2 : Delay  DelayLength=PI_params.delay_Currents
  Gain : Gain  Gain=pmsm.QEPSlits*4/(2*pi)  OutDataTypeStr=uint16  RndMeth=Simplest
  Get_ADC_Counts : Gain  Gain=2048  RndMeth=Simplest  OutDataTypeStr=Inherit: Same as input
  Get_PU : Gain  Gain=1/PU_System.I_base  RndMeth=Simplest
  Mod : Math  Operator=mod
  Mux : Mux  Inputs=2
  Saturation : Saturate  UpperLimit=2048  LowerLimit=-2048
  Saturation1 : Saturate  UpperLimit=4095  LowerLimit=0
  Selector : Selector  InputPortWidth=3  IndexOptions=Index vector (dialog)  Indices=[1 2]  OutputSizes=1
  Step : Step  Time=0.01  OutDataTypeStr=single  SampleTime=0
  ~1.65V in ADC counts : Constant  Value=[inverter.CtSensAOffset inverter.CtSensBOffset]  OutDataTypeStr=uint16  SampleTime=-1
  PhaseCurr_fb : Outport
  Position_fb : Outport  Port=2
  wires:
  Get_ADC_Counts/1 -> Saturation/1
  Saturation1/1 -> Data Type Conversion1/1
  Add4/1 -> Saturation1/1
  ~1.65V in ADC counts/1 -> Add4/2
  Delay1/1 -> Selector/1  "Iab_fb"
  Saturation/1 -> Add4/1
  Data Type Conversion4/1 -> Delay1/1
  Get_PU/1 -> Get_ADC_Counts/1
  Selector/1 -> Get_PU/1
  PhaseCurr/1 -> Data Type Conversion4/1
  Data Type Conversion2/1 -> Delay2/1
  Delay2/1 -> Mod/1
  Constant/1 -> Mod/2
  Mod/1 -> Gain/1
  Data Type Conversion1/1 -> PhaseCurr_fb/1
  Info/1 -> Data Type Conversion2/1
  Mux/1 -> Position_fb/1
  Gain/1 -> Mux/1
  Step/1 -> Data Type Conversion3/1
  Data Type Conversion3/1 -> Mux/2

== system mcb_microchip_pmsm_autotuner_SAME70/Microcontroller/Application/Current Control/Current_Controllers ==
  Id : Inport
  Iq : Inport  Port=2
  En : Inport  Port=3
  PIParams : Inport  Port=4
  Idq_Ref : Inport  Port=5
  Demux : Demux  Outputs=2
  En1 : InportShadow  Port=3
  Mux : Mux
  PIParams1 : InportShadow  Port=4
  PI_Controller_Id : Subsystem
  PI_Controller_Iq : Subsystem
  Vd_ref : Outport  VectorParamsAs1DForOutWhenUnconnected=off
  Vq_ref : Outport  Port=2  VectorParamsAs1DForOutWhenUnconnected=off
  Idq : Outport  Port=3  VectorParamsAs1DForOutWhenUnconnected=off
  wires:
  Iq/1 -> Mux/4, PI_Controller_Iq/2(I_fb)  "Iq_fb"
  Id/1 -> PI_Controller_Id/2(I_fb), Mux/2  "Id_fb"
  Demux/1 -> PI_Controller_Id/1(I_ref), Mux/1  "Id_Ref"
  Demux/2 -> Mux/3, PI_Controller_Iq/1(I_ref)  "Iq_Ref"
  Idq_Ref/1 -> Demux/1
  Mux/1 -> Idq/1
  PI_Controller_Id/1(V_ref) -> Vd_ref/1
  PI_Controller_Iq/1(V_ref) -> Vq_ref/1
  En/1 -> PI_Controller_Id/3(En)
  En1/1 -> PI_Controller_Iq/3(En)
  PIParams/1 -> PI_Controller_Id/4(PIParams)
  PIParams1/1 -> PI_Controller_Iq/4(PIParams)

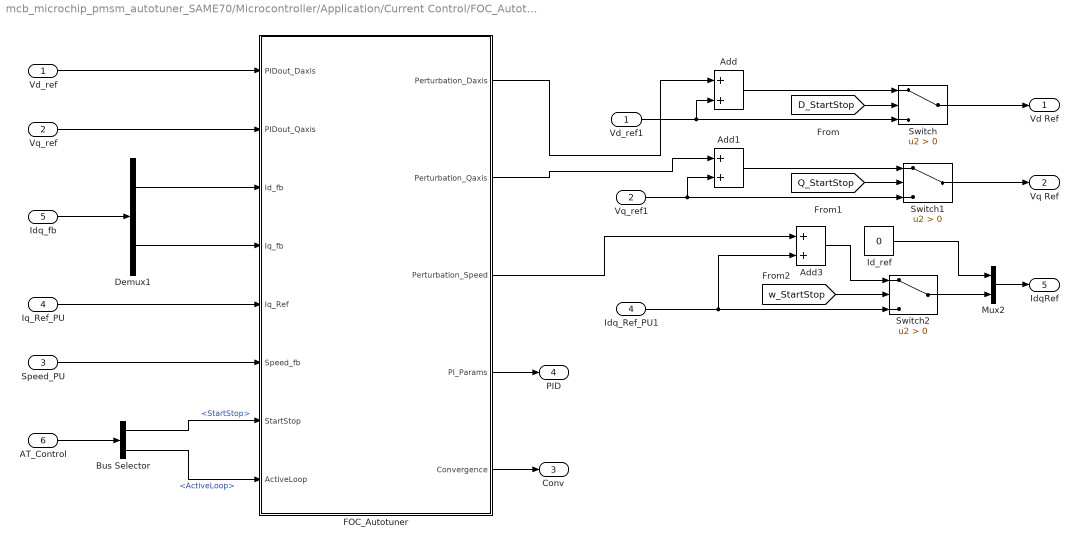
== system mcb_microchip_pmsm_autotuner_SAME70/Microcontroller/Application/Current Control/FOC_Autotuner ==
  Vd_ref : Inport
  Vq_ref : Inport  Port=2
  Speed_PU : Inport  Port=3
  Iq_Ref_PU : Inport  Port=4
  Idq_fb : Inport  Port=5
  AT_Control : Inport  Port=6
  Add : Sum
  Add1 : Sum
  Add3 : Sum
  Bus Selector : BusSelector  OutputSignals=StartStop,ActiveLoop
  Demux1 : Demux  Outputs=2
  FOC_Autotuner : Subsystem
  Id_ref : Constant  Value=0  OutDataTypeStr=dataType  SampleTime=Ts
  Idq_Ref_PU1 : InportShadow  Port=4
  Mux2 : Mux  Inputs=2
  Switch : Switch  Criteria=u2 > Threshold  SaturateOnIntegerOverflow=off  InputSameDT=off
  Switch1 : Switch  Criteria=u2 > Threshold  SaturateOnIntegerOverflow=off  InputSameDT=off
  Switch2 : Switch  Criteria=u2 > Threshold  SaturateOnIntegerOverflow=off  InputSameDT=off
  Vd_ref1 : InportShadow
  Vq_ref1 : InportShadow  Port=2
  Vd Ref : Outport
  Vq Ref : Outport  Port=2
  Conv : Outport  Port=3
  PID : Outport  Port=4
  IdqRef : Outport  Port=5
  wires:
  [w_StartStop] -> Switch2/2
  [Q_StartStop] -> Switch1/2
  [D_StartStop] -> Switch/2
  FOC_Autotuner/5(Convergence) -> Conv/1
  FOC_Autotuner/4(PI_Params) -> PID/1
  FOC_Autotuner/3(Perturbation_Speed) -> Add3/1
  FOC_Autotuner/2(Perturbation_Qaxis) -> Add1/1
  FOC_Autotuner/1(Perturbation_Daxis) -> Add/1
  Speed_PU/1 -> FOC_Autotuner/6(Speed_fb)
  Iq_Ref_PU/1 -> FOC_Autotuner/5(Iq_Ref)
  Demux1/2 -> FOC_Autotuner/4(Iq_fb)
  Vq_ref/1 -> FOC_Autotuner/2(PIDout_Qaxis)
  Demux1/1 -> FOC_Autotuner/3(Id_fb)
  Vd_ref/1 -> FOC_Autotuner/1(PIDout_Daxis)
  Idq_Ref_PU1/1 -> Switch2/3, Add3/2
  Add3/1 -> Switch2/1
  Switch2/1 -> Mux2/2
  Mux2/1 -> IdqRef/1
  Id_ref/1 -> Mux2/1
  Switch/1 -> Vd Ref/1
  Idq_fb/1 -> Demux1/1
  Vd_ref1/1 -> Add/2, Switch/3
  Vq_ref1/1 -> Add1/2, Switch1/3
  Switch1/1 -> Vq Ref/1
  Add/1 -> Switch/1
  Add1/1 -> Switch1/1
  AT_Control/1 -> Bus Selector/1
  Bus Selector/1 -> FOC_Autotuner/7(StartStop)  "<StartStop>"
  Bus Selector/2 -> FOC_Autotuner/8(ActiveLoop)  "<ActiveLoop>"

== system mcb_microchip_pmsm_autotuner_SAME70/Microcontroller/Application/Speed Control/PI_Controller_Speed ==
  N_ref : Inport
  N_fb : Inport  Port=2
  Enable : Inport  Port=3
  EnClosedLoop : Inport  Port=4
  PIParams : Inport  Port=5
  AND : Logic  IconShape=distinctive  AllPortsSameDT=off  OutDataTypeStr=boolean
  Bus Selector : BusSelector  OutputSignals=KpSpeed,KiSpeed
  Discrete PI Controller with anti-windup & reset : slpidlib/PID Controller  Controller=PI  Form=Parallel  TimeDomain=Discrete-time  UseExternalTs=off  SampleTime=-1  IntegratorMethod=Forward Euler  FilterMethod=Forward Euler  ControllerParametersSource=external  P=1  I=1  UseKiTs=on  D=0  N=100  UseFilter=on  TunerSelectOption=Transfer Function Based (PID Tuner App)  InitialConditionSource=external  InitialConditionForIntegrator=0  InitialConditionForFilter=0  DifferentiatorICPrevScaledInput=0  ExternalReset=level  TrackingMode=off  Kt=1  LimitOutput=on  SatLimitsSource=internal  UpperSaturationLimit=1  LowerSaturationLimit=-1  LinearizeAsGain=on  AntiWindupMode=clamping  Kb=1  LimitIntegrator=off  UpperIntegratorSaturationLimit=inf  LowerIntegratorSaturationLimit=-inf  RndMeth=Simplest  POutMin=[]  POutMax=[]  IOutMin=[]  IOutMax=[]  DOutMin=[]  DOutMax=[]  NOutMin=[]  NOutMax=[]  SumOutMin=[]  SumOutMax=[]  SaturationOutDataTypeStr=Inherit: Inherit via back propagation  SaturationOutMin=[]  SaturationOutMax=[]  PParamMin=[]  PParamMax=[]  IParamMin=[]  IParamMax=[]  DParamMin=[]  DParamMax=[]  NParamMin=[]  NParamMax=[]  KbParamMin=[]  KbParamMax=[]  KtParamMin=[]  KtParamMax=[]  KbOutMin=[]  KbOutMax=[]  KtOutMin=[]  KtOutMax=[]  IntegratorOutMin=[]  IntegratorOutMax=[]  FilterOutMin=[]  FilterOutMax=[]  SumI1OutMin=[]  SumI1OutMax=[]  SumI2OutMin=[]  SumI2OutMax=[]  SumI3OutMin=[]  SumI3OutMax=[]  SumI4OutMin=[]  SumI4OutMax=[]  SumDOutMin=[]  SumDOutMax=[]  DifferentiatorOutMin=[]  DifferentiatorOutMax=[]  FilterDiffOutCoefMin=[]  FilterDiffOutCoefMax=[]  ReciprocalOutMin=[]  ReciprocalOutMax=[]  SumDenOutMin=[]  SumDenOutMax=[]  SumNumOutMin=[]  SumNumOutMax=[]  DivideOutMin=[]  DivideOutMax=[]  UdiffTsProdOutMin=[]  UdiffTsProdOutMax=[]  NTsProdOutMin=[]  NTsProdOutMax=[]  UintegralTsProdOutMin=[]  UintegralTsProdOutMax=[]  UngainTsProdOutMin=[]  UngainTsProdOutMax=[]  ClampingZeroOutDataTypeStr=Inherit: Inherit via back propagation  ClampingZeroOutMin=[]  ClampingZeroOutMax=[]  FilterDenConstantOutDataTypeStr=Inherit: Inherit via back propagation  FilterDenConstantOutMin=[]  FilterDenConstantOutMax=[]  PCopyOutDataTypeStr=Inherit: Inherit via back propagation  PCopyOutMin=[]  PCopyOutMax=[]  NCopyOutDataTypeStr=Inherit: Inherit via back propagation  NCopyOutMin=[]  NCopyOutMax=[]  IntegratorContinuousStateAttributes=''  IntegratorStateMustResolveToSignalObject=off  IntegratorRTWStateStorageClass=Auto  FilterContinuousStateAttributes=''  FilterStateMustResolveToSignalObject=off  FilterRTWStateStorageClass=Auto  ParallelPVariant=ExternalParameters  IdealPVariant=Disabled  IVariant=ExternalParameters  DVariant=Disabled  IntegratorVariant=Discrete  SatVariant=Enabled  AWVariant=DiscClampingParallel  PCopyVariant=Disabled  TRVariant=Disabled  FdbkBlocksVariant=Forward  IdealPFdbkVariant=Disabled  SatFdbkVariant=Disabled  DerivativeFilterVariant=Disabled  NVariant=Disabled  NCopyVariant=Disabled_SignalSpec  FilterICVariant=Disabled  IntegratorICVariant=ExternalICs  ExternalResetVariant=ExternalReset  TRSumVariant=Passthrough  SumFdbkVariant=Disabled  SumVariant=Sum_PI  TsampFilterVariant=InternalTs  TsampNgainVariant=Passthrough  TsampIntegralVariant=Disabled_SignalSpec  ExternalSaturationOutDataTypeStr=Inherit: Same as second input
  Gain : Gain  Gain=Ts_speed
  Ki2 : Constant  Value=0  OutDataTypeStr=dataType  SampleTime=-1
  Logical Operator : Logic  Operator=NOT  IconShape=distinctive  AllPortsSameDT=off  OutDataTypeStr=boolean
  Sum : Sum  Inputs=|+-  OutDataTypeStr=Inherit: Same as first input
  Iq_ref : Outport  VectorParamsAs1DForOutWhenUnconnected=off
  wires:
  Bus Selector/1 -> Discrete PI Controller with anti-windup & reset/2  "<KpSpeed>"
  Bus Selector/2 -> Gain/1  "<KiSpeed>"
  Gain/1 -> Discrete PI Controller with anti-windup & reset/3
  AND/1 -> Logical Operator/1
  EnClosedLoop/1 -> AND/2
  Enable/1 -> AND/1
  Ki2/1 -> Discrete PI Controller with anti-windup & reset/5
  Logical Operator/1 -> Discrete PI Controller with anti-windup & reset/4
  Sum/1 -> Discrete PI Controller with anti-windup & reset/1
  N_ref/1 -> Sum/1
  N_fb/1 -> Sum/2
  Discrete PI Controller with anti-windup & reset/1 -> Iq_ref/1
  PIParams/1 -> Bus Selector/1

== system mcb_microchip_pmsm_autotuner_SAME70/Microcontroller/Application Abstraction/Variant Subsystem/Index Absent ==
  eQEPCnt : Inport
  eQEPIndex : Inport  Port=2
  Mode : Inport  Port=3
  Compare To Constant : simulink/Logic and Bit Operations/Compare To Constant  relop=>=  const=2  OutDataTypeStr=boolean
  Compare To Constant1 : simulink/Logic and Bit Operations/Compare To Constant  relop=<  const=2  OutDataTypeStr=boolean
  Enabled Subsystem : Subsystem  TreatAsAtomicUnit=on
  IIR Filter4 : mcbcontrolslib/IIR Filter  VariantControl=Low Pass Filter  VariantSelect=Low-pass  Filter_constant=0.01  advancedSettings=off  Ts=50e-6  cutOff_freq=32.1525
  Mechanical to Electrical Position : mcbpositiondecoderlib/Mechanical to Electrical Position  NrPP=pmsm.p  selectedRange=Radians  MechOfstInputType=Input port  mechOffsetIn=0  maxAngleIn=2*pi  InputDataType=dataType  VariantSelect=floating-point
  Quadrature Decoder : mcbpositiondecoderlib/Quadrature Decoder  EncoderSlitsPerRevolution=pmsm.QEPSlits  EncoderCountsPerSlit=4  CounterSize=16 bits  ExternalIndexCount=off  PositionUnit=Radians  PositionDataType=dataType
  Speed Measurement : mcbpositiondecoderlib/Speed Measurement  PositionUnit=Radians  PositionScalingDatatype=uint32  SpeedCalculationMode=Time interval for speed calculation  SampleTimeAsync=Ts  MaximumApplicationSpeed=60000  SpeedResolution=5e-6  DelayLength=20  MaximumMeasurableSpeed=29999  MeasurableSpeedResolution=1.397e-05  SpeedUnit=RPM  PerUnitSpeed=PU_System.N_base  SpeedDataType=dataType
  Terminator : Terminator
  Theta : Outport
  Speed : Outport  Port=2
  EnClosedLoop : Outport  Port=3
  wires:
  eQEPIndex/1 -> Terminator/1
  Compare To Constant/1 -> EnClosedLoop/1
  Mode/1 -> Compare To Constant1/1, Compare To Constant/1
  eQEPCnt/1 -> Quadrature Decoder/1
  Quadrature Decoder/1 -> Speed Measurement/1, Enabled Subsystem/1(In1), Mechanical to Electrical Position/1
  Mechanical to Electrical Position/1 -> Theta/1
  Compare To Constant1/1 -> Enabled Subsystem/Enable
  Enabled Subsystem/1(Out1) -> Mechanical to Electrical Position/2
  Speed Measurement/1 -> IIR Filter4/1
  IIR Filter4/1 -> Speed/1

== system mcb_microchip_pmsm_autotuner_SAME70/Microcontroller/Application Abstraction/Variant Subsystem/Index Present ==
  eQEPCnt : Inport
  eQEPIndex : Inport  Port=2
  Mode : Inport  Port=3
  Theta : Outport
  Speed : Outport  Port=2
  EnClosedLoop : Outport  Port=3

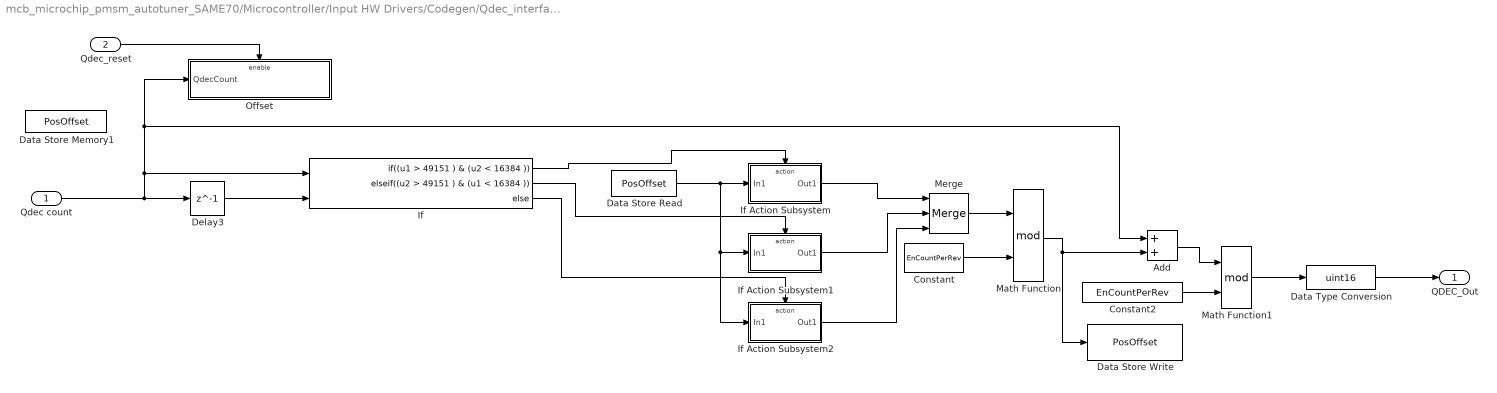
== system mcb_microchip_pmsm_autotuner_SAME70/Microcontroller/Input HW Drivers/Codegen/Qdec_interface ==
  Qdec count : Inport
  Qdec_reset : Inport  Port=2  OutDataTypeStr=boolean
  Add : Sum  OutDataTypeStr=single
  Constant : Constant  Value=EnCountPerRev  OutDataTypeStr=Inherit: Inherit via back propagation
  Constant2 : Constant  Value=EnCountPerRev  OutDataTypeStr=Inherit: Inherit via back propagation
  Data Store Memory1 : DataStoreMemory  DataStoreName=PosOffset  ShowAdditionalParam=off  OutDataTypeStr=uint16
  Data Store Read : DataStoreRead  DataStoreName=PosOffset  IndexOptions=Index vector (dialog)  Indices=1  OutputSizes=1
  Data Store Write : DataStoreWrite  DataStoreName=PosOffset  IndexOptions=Index vector (dialog)  Indices=1  OutputSizes=1
  Data Type Conversion : DataTypeConversion  OutDataTypeStr=uint16  SaturateOnIntegerOverflow=off  RndMeth=Floor
  Delay3 : Delay  DelayLength=1  InitialCondition=0
  If : If  NumInputs=2  IfExpression=(u1 > 49151 ) & (u2 < 16384 )  ElseIfExpressions=(u2 > 49151 ) & (u1 < 16384 )
  If Action Subsystem : Subsystem  TreatAsAtomicUnit=on
  If Action Subsystem1 : Subsystem  TreatAsAtomicUnit=on
  If Action Subsystem2 : Subsystem  TreatAsAtomicUnit=on
  Math Function : Math  Operator=mod  SignedPower=on
  Math Function1 : Math  Operator=mod  SignedPower=on
  Merge : Merge  Inputs=3
  Offset : Subsystem
  QDEC_Out : Outport
  wires:
  Qdec count/1 -> Offset/1(QdecCount), Add/1, If/1, Delay3/1
  If Action Subsystem2/1(Out1) -> Merge/3
  If/2 -> If Action Subsystem1/Action
  If Action Subsystem1/1(Out1) -> Merge/2
  Data Store Read/1 -> If Action Subsystem2/1(In1), If Action Subsystem1/1(In1), If Action Subsystem/1(In1)
  If/3 -> If Action Subsystem2/Action
  If Action Subsystem/1(Out1) -> Merge/1
  Constant/1 -> Math Function/2
  Delay3/1 -> If/2
  Merge/1 -> Math Function/1
  If/1 -> If Action Subsystem/Action
  Math Function/1 -> Data Store Write/1, Add/2
  Add/1 -> Math Function1/1
  Constant2/1 -> Math Function1/2
  Math Function1/1 -> Data Type Conversion/1
  Qdec_reset/1 -> Offset/Enable
  Data Type Conversion/1 -> QDEC_Out/1
